simulink model "prelab1b"  (Simulink 7.8)
settings: Solver=ode45  StartTime=0.0  StopTime=10.0  RelTol=1e-3
settings Model: Creator=Embed_Sys_course  LastModifiedBy=Embed_Sys_course

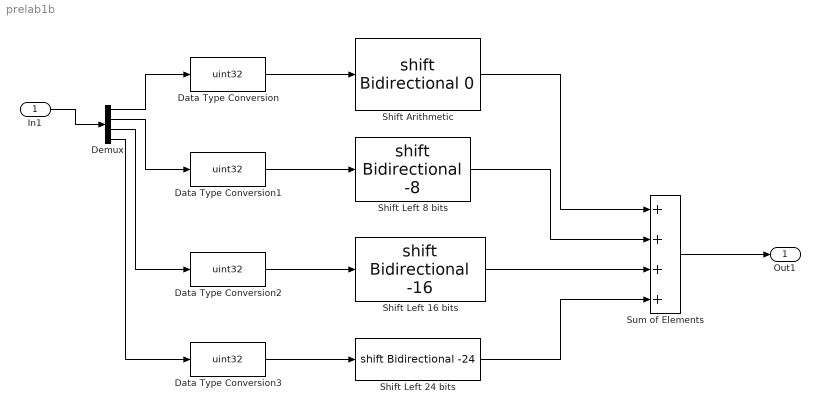
== system prelab1b ==
  In1 : Inport
  Data Type Conversion{,1..3} (4 alike) : DataTypeConversion  OutDataTypeStr=uint32
  Demux : Demux
  Shift Arithmetic : ArithShift
  Shift Left 16 bits : ArithShift  BitShiftNumber=-16
  Shift Left 24 bits : ArithShift  BitShiftNumber=-24
  Shift Left 8 bits : ArithShift  BitShiftNumber=-8
  Sum of Elements : Sum  Inputs=++++
  Out1 : Outport
  wires:
  In1/1 -> Demux/1
  Sum of Elements/1 -> Out1/1
  Data Type Conversion/1 -> Shift Arithmetic/1
  Data Type Conversion1/1 -> Shift Left 8 bits/1
  Data Type Conversion2/1 -> Shift Left 16 bits/1
  Data Type Conversion3/1 -> Shift Left 24 bits/1
  Demux/1 -> Data Type Conversion/1
  Demux/2 -> Data Type Conversion1/1
  Demux/3 -> Data Type Conversion2/1
  Demux/4 -> Data Type Conversion3/1
  Shift Arithmetic/1 -> Sum of Elements/1
  Shift Left 8 bits/1 -> Sum of Elements/2
  Shift Left 16 bits/1 -> Sum of Elements/3
  Shift Left 24 bits/1 -> Sum of Elements/4
